simulink library "Navigation_Lib"  (R2014a)
settings: Solver=ode45  StartTime=0.0  StopTime=10.0  RelTol=1e-3
undefined symbols (not defined in the file or in its folder): DiscIntNeverNeededParam, gyro_x_offset, gyro_y_offset, gyro_z_offset
libraries: simulink x7, aerolibutil x5, vrlib x4, aerolibtransform2 x3, dspmtrx3 x2
(part 1 of 3)
settings Model: Creator=darenlee  LastModifiedBy=darenlee

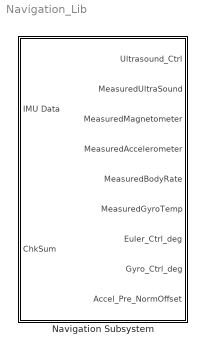
== system Navigation_Lib ==
  Navigation Subsystem : Subsystem  mask{TempProcessVariant=1, PI_YAW_CORRECT=[-0.9 -0.0001], D_YAW_CORRECT=0, P_GAIN_ROLLPITCH=-2, I_GAIN_ROLLPITCH=-0.01, ACCEL_OFFSET_X=0, ACCEL_OFFSET_Y=0, ACCEL_OFFSET_Z=0}
      mask prompts: TempProcessVariant "TempCondition"; PI_YAW_CORRECT "PI Gain  (Yaw Correction)"; D_YAW_CORRECT "D Gain (Yaw Correction)"; P_GAIN_ROLLPITCH "P Gain (RollPitch Correction)"; I_GAIN_ROLLPITCH "I Gain (RollPitch Correction)"; ACCEL_OFFSET_X "Accel Offset X"; ACCEL_OFFSET_Y "Accel Offset Y"; ACCEL_OFFSET_Z "Accel Offset Z"
      mask TypeOptions TempProcessVariant: 1 | 2
      mask DialogControl DescTextVar Prompt: Navigation Subsystem with Attitude Determination

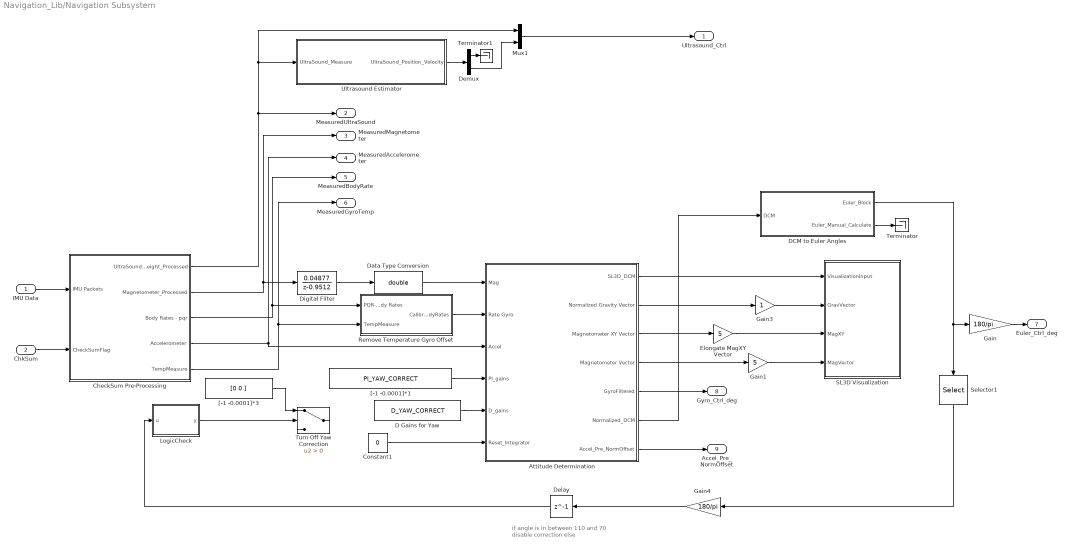
== system Navigation_Lib/Navigation Subsystem ==
  note: if angle is in between 110 and 70
      | disable correction
      | else
  IMU Data : Inport  OutDataTypeStr=Bus: IMU_Packets
  ChkSum : Inport  Port=2
  Attitude Determination : Subsystem
  CheckSum Pre-Processing : Subsystem
  Constant1 : Constant  Value=0
  D Gains for Yaw : Constant  Value=D_YAW_CORRECT
  DCM to Euler Angles : Subsystem
  Data Type Conversion : DataTypeConversion  OutDataTypeStr=double
  Delay : Delay  DelayLength=1  InitialCondition=0
  Demux : Demux  Outputs=2
  Digital Filter : DiscreteTransferFcn  Numerator=[0.04877]  Denominator=[1 -0.9512]  SampleTime=1/400
  Elongate MagXY Vector : Gain  Gain=5  OutDataTypeStr=double
  Gain : Gain  Gain=180/pi
  Gain1 : Gain  Gain=5  OutDataTypeStr=double
  Gain3 : Gain  OutDataTypeStr=double
  Gain4 : Gain  Gain=180/pi
  LogicCheck : MATLAB Function  TreatAsAtomicUnit=on
  Mux1 : Mux  Inputs=2
  Remove Temperature Gyro Offset : Subsystem  Variant=on  OverrideUsingVariant=TempProcessVariant==1
  SL3D Visualization : Subsystem
  Selector1 : Selector  IndexMode=Zero-based  InputPortWidth=3  Indices=2
  Terminator : Terminator
  Terminator1 : Terminator
  "Turn Off Yaw Correction " : Switch  Criteria=u2 > Threshold
  Ultrasound Estimator : Subsystem
  "[-1 -0.0001]*1" : Constant  Value=PI_YAW_CORRECT
  "[-1 -0.0001]*3" : Constant  Value=[0 0 ]
  Ultrasound_Ctrl : Outport
  MeasuredUltraSound : Outport  Port=2
  MeasuredMagnetometer : Outport  Port=3
  MeasuredAccelerometer : Outport  Port=4
  MeasuredBodyRate : Outport  Port=5
  MeasuredGyroTemp : Outport  Port=6
  Euler_Ctrl_deg : Outport  Port=7
  Gyro_Ctrl_deg : Outport  Port=8
  "Accel_Pre_NormOffset " : Outport  Port=9
  wires:
  DCM to Euler Angles/2(Euler_Manual_Calculate) -> Terminator/1
  "[-1 -0.0001]*1"/1 -> Attitude Determination/4(PI_gains)
  Remove Temperature Gyro Offset/1(Calibrated-BodyRates) -> Attitude Determination/2(Rate Gyro)
  D Gains for Yaw/1 -> Attitude Determination/5(D_gains)
  Gain4/1 -> Delay/1
  Selector1/1 -> Gain4/1
  LogicCheck/1(y) -> "Turn Off Yaw Correction "/2
  Delay/1 -> LogicCheck/1(u)
  "[-1 -0.0001]*3"/1 -> "Turn Off Yaw Correction "/1
  Attitude Determination/5(GyroFiltered) -> Gyro_Ctrl_deg/1
  Attitude Determination/3(" Magnetometer XY Vector") -> Elongate MagXY Vector/1
  Attitude Determination/4(Magnetometer Vector) -> Gain1/1
  Gain3/1 -> SL3D Visualization/2(GravVector)
  Attitude Determination/2(Normalized Gravity Vector) -> Gain3/1
  Constant1/1 -> Attitude Determination/6(Reset_Integrator)
  Elongate MagXY Vector/1 -> SL3D Visualization/3(MagXY)
  Gain1/1 -> SL3D Visualization/4(MagVector)
  Attitude Determination/1(SL3D_DCM) -> SL3D Visualization/1(VisualizationInput)
  Digital Filter/1 -> Data Type Conversion/1
  DCM to Euler Angles/1(Euler_Block) -> Gain/1, Selector1/1
  CheckSum Pre-Processing/5(TempMeasure) -> Remove Temperature Gyro Offset/2(TempMeasure), MeasuredGyroTemp/1
  CheckSum Pre-Processing/2(Magnetometer_Processed) -> Digital Filter/1, MeasuredMagnetometer/1
  CheckSum Pre-Processing/3(Body Rates - pqr) -> Remove Temperature Gyro Offset/1(PQR-Body Rates), MeasuredBodyRate/1
  CheckSum Pre-Processing/4(Accelerometer) -> Attitude Determination/3(Accel), MeasuredAccelerometer/1
  ChkSum/1 -> CheckSum Pre-Processing/2(CheckSumFlag)
  IMU Data/1 -> CheckSum Pre-Processing/1(IMU Packets)
  Attitude Determination/6("Normalized_DCM ") -> DCM to Euler Angles/1(DCM)
  Data Type Conversion/1 -> Attitude Determination/1(Mag)
  Attitude Determination/7(Accel_Pre_NormOffset) -> "Accel_Pre_NormOffset "/1
  Gain/1 -> Euler_Ctrl_deg/1
  CheckSum Pre-Processing/1(UltraSoundHeight_Processed) -> Ultrasound Estimator/1(UltraSound_Measure), Mux1/1, MeasuredUltraSound/1
  Mux1/1 -> Ultrasound_Ctrl/1
  Ultrasound Estimator/1("UltraSound_Position_Velocity ") -> Demux/1
  Demux/2 -> Mux1/2
  Demux/1 -> Terminator1/1

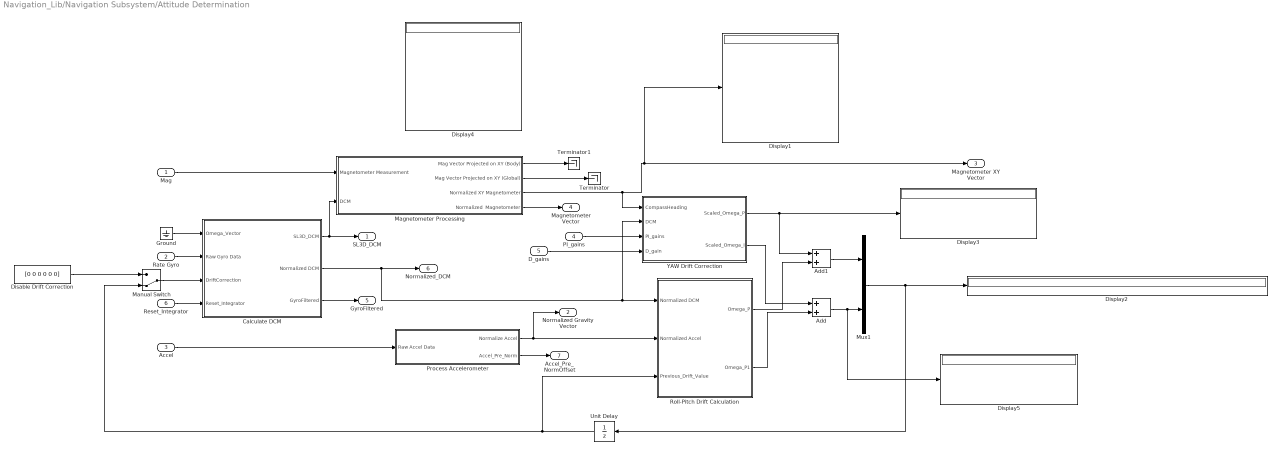
== system Navigation_Lib/Navigation Subsystem/Attitude Determination ==
  Mag : Inport  PortDimensions=3
  Rate Gyro : Inport  Port=2  PortDimensions=3
  Accel : Inport  Port=3  OutDataTypeStr=uint16
  PI_gains : Inport  Port=4
  D_gains : Inport  Port=5
  Reset_Integrator : Inport  Port=6
  Add : Sum
  Add1 : Sum
  Calculate DCM : Subsystem
  Disable Drift Correction : Constant  Value=[0 0 0 0 0 0]
  Display{1..5} (5 alike) : Display
  Ground : Ground
  Magnetometer Processing : Subsystem
  Manual Switch : ManualSwitch  CurrentSetting=0
  Mux1 : Mux  Inputs=2
  Process Accelerometer : Subsystem
  Roll-Pitch Drift Calculation : Subsystem
  Terminator : Terminator
  Terminator1 : Terminator
  Unit Delay : UnitDelay  SampleTime=-1
  YAW Drift Correction : Subsystem  TreatAsAtomicUnit=on
  SL3D_DCM : Outport
  Normalized Gravity Vector : Outport  Port=2
  " Magnetometer XY Vector" : Outport  Port=3
  Magnetometer Vector : Outport  Port=4
  GyroFiltered : Outport  Port=5
  "Normalized_DCM " : Outport  Port=6
  Accel_Pre_NormOffset : Outport  Port=7
  wires:
  Calculate DCM/2(Normalized DCM) -> YAW Drift Correction/2(DCM), Roll-Pitch Drift Calculation/1(Normalized DCM), "Normalized_DCM "/1
  Manual Switch/1 -> Calculate DCM/3(DriftCorrection)
  Process Accelerometer/1(Normalize Accel) -> Normalized Gravity Vector/1, Roll-Pitch Drift Calculation/2(Normalized Accel)
  D_gains/1 -> YAW Drift Correction/4(D_gain)
  Magnetometer Processing/1(Mag Vector Projected on XY (Body)) -> Terminator1/1
  Disable Drift Correction/1 -> Manual Switch/1
  Accel/1 -> Process Accelerometer/1(Raw Accel Data)
  Process Accelerometer/2(Accel_Pre_Norm) -> Accel_Pre_NormOffset/1
  Mag/1 -> Magnetometer Processing/1(Magnetometer Measurement)
  Magnetometer Processing/2(Mag Vector Projected on XY (Global)) -> Terminator/1
  Calculate DCM/1(SL3D_DCM) -> SL3D_DCM/1, Magnetometer Processing/2(DCM)
  Add/1 -> Display5/1, Mux1/2
  Add1/1 -> Mux1/1
  Roll-Pitch Drift Calculation/1(Omega_P) -> Add1/2
  Roll-Pitch Drift Calculation/2(Omega_P1) -> Add/2
  PI_gains/1 -> YAW Drift Correction/3(PI_gains)
  Magnetometer Processing/3(Normalized XY Magnetometer) -> Display1/1, " Magnetometer XY Vector"/1, YAW Drift Correction/1(CompassHeading)
  Magnetometer Processing/4(Normalized  Magnetometer) -> Magnetometer Vector/1
  YAW Drift Correction/1(Scaled_Omega_P) -> Display3/1, Add1/1
  YAW Drift Correction/2(Scaled_Omega_I) -> Add/1
  Reset_Integrator/1 -> Calculate DCM/4("Reset_Integrator ")
  Calculate DCM/3(GyroFiltered) -> GyroFiltered/1
  Mux1/1 -> Unit Delay/1, Display2/1
  Rate Gyro/1 -> Calculate DCM/2(Raw Gyro Data)
  Unit Delay/1 -> Manual Switch/2, Roll-Pitch Drift Calculation/3(Previous_Drift_Value)
  Ground/1 -> Calculate DCM/1(Omega_Vector)

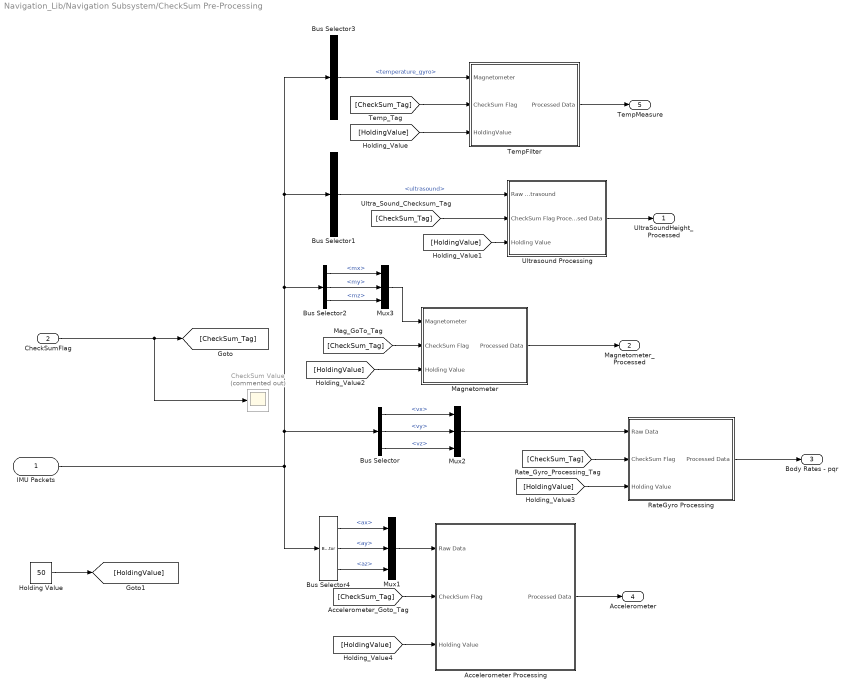
== system Navigation_Lib/Navigation Subsystem/CheckSum Pre-Processing ==
  IMU Packets : Inport
  CheckSumFlag : Inport  Port=2
  Accelerometer Processing : Subsystem
  Bus Selector : BusSelector  OutputSignals=vx,vy,vz
  Bus Selector1 : BusSelector  OutputSignals=ultrasound
  Bus Selector2 : BusSelector  OutputSignals=mx,my,mz
  Bus Selector3 : BusSelector  OutputSignals=temperature_gyro
  Bus Selector4 : BusSelector  OutputSignals=ax,ay,az
  CheckSum Value : Scope  Commented=on
      settings: YMin=0  YMax=2500  SaveName=CheckSum
  Holding Value : Constant  Value=50
  Magnetometer : Subsystem
  Mux1 : Mux  Inputs=3
  Mux2 : Mux  Inputs=3
  Mux3 : Mux  Inputs=3
  RateGyro Processing : Subsystem
  TempFilter : Subsystem
  Ultrasound Processing : Subsystem
  UltraSoundHeight_Processed : Outport
  Magnetometer_Processed : Outport  Port=2
  Body Rates - pqr : Outport  Port=3
  Accelerometer : Outport  Port=4
  TempMeasure : Outport  Port=5
  wires:
  Holding Value/1 -> [HoldingValue]
  [HoldingValue] -> Accelerometer Processing/3(Holding Value)
  [HoldingValue] -> RateGyro Processing/3(Holding Value)
  [HoldingValue] -> Magnetometer/3(Holding Value)
  [HoldingValue] -> Ultrasound Processing/3(Holding Value)
  [HoldingValue] -> TempFilter/3(HoldingValue)
  [CheckSum_Tag] -> TempFilter/2(CheckSum Flag)
  TempFilter/1(Processed Data) -> TempMeasure/1
  Bus Selector3/1 -> TempFilter/1(Magnetometer)  "<temperature_gyro>"
  Bus Selector/3 -> Mux2/3  "<vz>"
  Bus Selector/2 -> Mux2/2  "<vy>"
  Bus Selector/1 -> Mux2/1  "<vx>"
  Ultrasound Processing/1(Processed Data) -> UltraSoundHeight_Processed/1
  [CheckSum_Tag] -> Accelerometer Processing/2(CheckSum Flag)
  Magnetometer/1(Processed Data) -> Magnetometer_Processed/1
  [CheckSum_Tag] -> Magnetometer/2(CheckSum Flag)
  Mux3/1 -> Magnetometer/1(Magnetometer)
  Bus Selector2/3 -> Mux3/3  "<mz>"
  Bus Selector2/2 -> Mux3/2  "<my>"
  Bus Selector2/1 -> Mux3/1  "<mx>"
  RateGyro Processing/1(Processed Data) -> Body Rates - pqr/1
  [CheckSum_Tag] -> RateGyro Processing/2(CheckSum Flag)
  Mux2/1 -> RateGyro Processing/1(Raw Data)
  Accelerometer Processing/1(Processed Data) -> Accelerometer/1
  [CheckSum_Tag] -> Ultrasound Processing/2(CheckSum Flag)
  Mux1/1 -> Accelerometer Processing/1(Raw Data)
  Bus Selector4/3 -> Mux1/3  "<az>"
  Bus Selector4/2 -> Mux1/2  "<ay>"
  Bus Selector4/1 -> Mux1/1  "<ax>"
  IMU Packets/1 -> Bus Selector4/1, Bus Selector2/1, Bus Selector1/1, Bus Selector3/1, Bus Selector/1
  CheckSumFlag/1 -> CheckSum Value/1, [CheckSum_Tag]
  Bus Selector1/1 -> Ultrasound Processing/1(Raw Ultrasound)  "<ultrasound>"

== system Navigation_Lib/Navigation Subsystem/DCM to Euler Angles ==
  note: Euler Rotation Order:
      | With the camera facing towards you
      | ______________
      |       Camera          |
      | 1                    2    |
      |                             |
      | 3                    4    |
      | ______________|
      |
      | Rotation
      |
      | Roll+ , increase 2+4
      | Roll - , increase 1 3
      |
      | Pitch+ , increaes 1+2
      | Pitch- , increase 3+4
  DCM : Inport
  Constant2 : Constant  Value=[1 0 0]
  Direction Cosine Matrix to Rotation Angles : aerolibtransform2/Direction Cosine Matrix to Rotation Angles  rotationOrder=XYZ  lim=Default
      settings: AttributesFormatString=Rotation Order: %<rotationOrder>
  EulerAnglesCalculation : Subsystem  TreatAsAtomicUnit=on
  Product : Product  Multiplication=Matrix(*)
  VectorTrace : Scope
      settings: SaveName=RotationVectorTrace
  Euler_Block : Outport
  Euler_Manual_Calculate : Outport  Port=2
  wires:
  Product/1 -> VectorTrace/1
  Constant2/1 -> Product/2
  Direction Cosine Matrix to Rotation Angles/1 -> Euler_Block/1
  EulerAnglesCalculation/1(Euler Angles) -> Euler_Manual_Calculate/1
  DCM/1 -> EulerAnglesCalculation/1(DCM), Product/1, Direction Cosine Matrix to Rotation Angles/1

== system Navigation_Lib/Navigation Subsystem/Remove Temperature Gyro Offset ==
  note: 1) Only subsystems can be added as variant choices at this level
      | 2) Blocks cannot be connected at this level as connectivity is
      | automatically determined at simulation, based on the active variant
  PQR-Body Rates : Inport
  TempMeasure : Inport  Port=2
  TemperatureOffset (home_330453) : Subsystem  VariantControl=TempProcessVariant==1
  TemperatureOffset (work_255725) : Subsystem  VariantControl=TempProcessVariant==2
  Calibrated-BodyRates : Outport

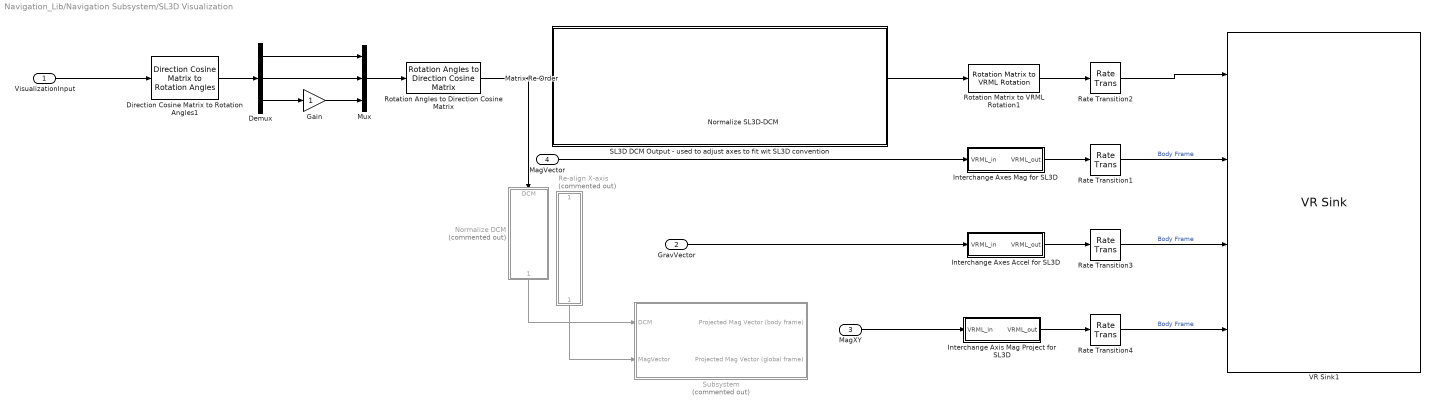
== system Navigation_Lib/Navigation Subsystem/SL3D Visualization ==
  VisualizationInput : Inport
  GravVector : Inport  Port=2
  MagXY : Inport  Port=3
  MagVector : Inport  Port=4
  Demux : Demux  Outputs=3
  Direction Cosine Matrix to Rotation Angles1 : aerolibtransform2/Direction Cosine Matrix to Rotation Angles  rotationOrder=XYZ  lim=ZeroR3
      settings: AttributesFormatString=Rotation Order: %<rotationOrder>
  Gain : Gain  OutDataTypeStr=Inherit: Same as input
  "Interchange Axes Accel for SL3D " : Subsystem
  "Interchange Axes Mag for SL3D " : Subsystem
  Interchange Axis Mag Project for SL3D : Subsystem
  Matrix Re-Order : MATLAB Function  TreatAsAtomicUnit=on
  Mux : Mux  Inputs=3
  Normalize DCM : Subsystem  Commented=on  TreatAsAtomicUnit=on
  Normalize SL3D-DCM : Subsystem  TreatAsAtomicUnit=on
  Rate Transition{1..4} (4 alike) : RateTransition
  Re-align X-axis : Subsystem  Commented=on
  Rotation Angles to Direction Cosine Matrix : aerolibtransform2/Rotation Angles to Direction Cosine Matrix  rotationOrder=XYZ
  Rotation Matrix to VRML Rotation1 : vrlib/Utilities/Rotation Matrix to VRML Rotation  maxzero=1e-12
  SL3D DCM Output - used to adjust axes to fit wit SL3D convention : Subsystem
  Subsystem : Subsystem  Commented=on
  VR Sink1 : vrlib/VR Sink  InstantiateOnLoad=on  SampleTime=0.02  ViewEnable=on  RemoteChange=off  RemoteView=off  FieldsWritten=Plane.rotation.4.1.1.double#mag_point.translation.3.1.1.double#grav_point.translation.3.1.1.double#mag_projection_point.translation.3.1.1.double  WorldFileName=AR_Drone_Visualization.WRL  AutoView=off  VideoDimensions=[]  AllowVariableSize=off
  wires:
  MagXY/1 -> Interchange Axis Mag Project for SL3D/1(VRML_in)
  Re-align X-axis/1(MagVectorOut) -> Subsystem/2(MagVector)
  Normalize DCM/1(DCM_normalized) -> Subsystem/1(DCM)
  Rate Transition2/1 -> VR Sink1/1
  Rate Transition1/1 -> VR Sink1/2  "Body Frame"
  Rate Transition3/1 -> VR Sink1/3  "Body Frame"
  Rate Transition4/1 -> VR Sink1/4  "Body Frame"
  Interchange Axis Mag Project for SL3D/1(VRML_out) -> Rate Transition4/1
  Rotation Angles to Direction Cosine Matrix/1 -> Normalize DCM/1(DCM), Matrix Re-Order/1(M_in)
  MagVector/1 -> "Interchange Axes Mag for SL3D "/1(VRML_in)
  "Interchange Axes Mag for SL3D "/1(VRML_out) -> Rate Transition1/1
  Normalize SL3D-DCM/1(DCM_normalized) -> Rotation Matrix to VRML Rotation1/1
  Matrix Re-Order/1(M_out) -> Normalize SL3D-DCM/1(DCM)
  GravVector/1 -> "Interchange Axes Accel for SL3D "/1(VRML_in)
  "Interchange Axes Accel for SL3D "/1(VRML_out) -> Rate Transition3/1
  Rotation Matrix to VRML Rotation1/1 -> Rate Transition2/1
  Direction Cosine Matrix to Rotation Angles1/1 -> Demux/1
  Demux/1 -> Mux/1
  Demux/2 -> Mux/2
  Demux/3 -> Gain/1
  Gain/1 -> Mux/3
  Mux/1 -> Rotation Angles to Direction Cosine Matrix/1
  VisualizationInput/1 -> Direction Cosine Matrix to Rotation Angles1/1

== system Navigation_Lib/Navigation Subsystem/Ultrasound Estimator ==
  UltraSound_Measure : Inport
  Kalman Tracker : MATLAB Function  TreatAsAtomicUnit=on
  Unit Delay1 : UnitDelay  InitialCondition=[0 0 ]  SampleTime=-1
  Unit Delay2 : UnitDelay  InitialCondition=eye(2)  SampleTime=-1
  "UltraSound_Position_Velocity " : Outport
  wires:
  Kalman Tracker/2(covariance_correction) -> Unit Delay2/1
  Kalman Tracker/1(state_correction) -> Unit Delay1/1
  UltraSound_Measure/1 -> Kalman Tracker/1(UltraSoundMeasure)
  Unit Delay2/1 -> Kalman Tracker/2(covariance_correction_input)
  Unit Delay1/1 -> "UltraSound_Position_Velocity "/1, Kalman Tracker/3(state_correction_input)

== system Navigation_Lib/Navigation Subsystem/Attitude Determination/Calculate DCM ==
  Omega_Vector : Inport
  Raw Gyro Data : Inport  Port=2
  DriftCorrection : Inport  Port=3
  "Reset_Integrator " : Inport  Port=4
  Calculate Deltas : Subsystem
  Matrix Re-Order : MATLAB Function  Commented=through  TreatAsAtomicUnit=on
  Normalize DCM : Subsystem  TreatAsAtomicUnit=on
  Normalize SL3D-DCM : Subsystem  Commented=through  TreatAsAtomicUnit=on
  Process Raw Rate Gyro Data : Subsystem
  SL3D DCM Output - used to adjust axes to fit wit SL3D convention : Subsystem
  Terminator : Terminator
  Update DCM : Subsystem  TreatAsAtomicUnit=on  VariantControl=UncorrectedMode
  deg2rad : Gain  Gain=pi/180
  SL3D_DCM : Outport
  Normalized DCM : Outport  Port=2
  GyroFiltered : Outport  Port=3
  wires:
  Process Raw Rate Gyro Data/1(Processed Data) -> deg2rad/1
  deg2rad/1 -> Calculate Deltas/1(Adjusted)
  Calculate Deltas/2(Omega) -> GyroFiltered/1, Terminator/1
  Raw Gyro Data/1 -> Process Raw Rate Gyro Data/1(Raw Data)
  Update DCM/1(DCM Matrix) -> Matrix Re-Order/1(M_in), Normalize DCM/1(DCM)
  Normalize DCM/1(DCM_normalized) -> Normalized DCM/1
  Omega_Vector/1 -> Update DCM/1(Omega vector)
  Calculate Deltas/1(Gyro_Vector(G_Dt)) -> Update DCM/2(Gyro vector)
  Matrix Re-Order/1(M_out) -> Normalize SL3D-DCM/1(DCM)
  Normalize SL3D-DCM/1(DCM_normalized) -> SL3D_DCM/1
  DriftCorrection/1 -> Calculate Deltas/2(DriftCorrection)
  "Reset_Integrator "/1 -> Update DCM/3("Reset_Integrator ")

== system Navigation_Lib/Navigation Subsystem/Attitude Determination/Magnetometer Processing ==
  Magnetometer Measurement : Inport
  DCM : Inport  Port=2
  Magnetometer Heading Calculation : Subsystem
  Normalize Vector : vrlib/Utilities/Normalize Vector  maxzero=0
  Normalize Vector1 : vrlib/Utilities/Normalize Vector  maxzero=0
  Process Raw Mag Data : Subsystem  Variant=on  OverrideUsingVariant=TempProcessVariant==1
  Re-align X-axis : Subsystem
  Mag Vector Projected on XY (Body) : Outport
  Mag Vector Projected on XY (Global) : Outport  Port=2
  Normalized XY Magnetometer : Outport  Port=3
  Normalized  Magnetometer : Outport  Port=4
  wires:
  Magnetometer Heading Calculation/2(Projected Mag Vector (global frame)) -> Mag Vector Projected on XY (Global)/1
  Normalize Vector/1 -> Normalized  Magnetometer/1, Re-align X-axis/1(MagVector)
  Process Raw Mag Data/1(MagVector) -> Normalize Vector/1
  Re-align X-axis/1(MagVectorOut) -> Magnetometer Heading Calculation/1(MagVector)
  Magnetometer Measurement/1 -> Process Raw Mag Data/1(Magnetometer)
  Magnetometer Heading Calculation/1(Projected Mag Vector (body frame)) -> Normalize Vector1/1
  DCM/1 -> Magnetometer Heading Calculation/2(DCM)
  Normalize Vector1/1 -> Normalized XY Magnetometer/1, Mag Vector Projected on XY (Body)/1

== system Navigation_Lib/Navigation Subsystem/Attitude Determination/Process Accelerometer ==
  Raw Accel Data : Inport
  Accelerometer Correction Offset : Subsystem
  Accelerometer Neutral Gain and Offset : Subsystem
  Low Pass Filter : Subsystem
  Normalize Accel : Outport
  Accel_Pre_Norm : Outport  Port=2
  wires:
  Raw Accel Data/1 -> Accelerometer Neutral Gain and Offset/1(Raw Accel Data)
  Accelerometer Neutral Gain and Offset/2(Accel_Pre_Norm) -> Accel_Pre_Norm/1
  Accelerometer Neutral Gain and Offset/1(Processed Accel Data) -> Accelerometer Correction Offset/1(Accelerometer)
  Accelerometer Correction Offset/1(OffsetCorrection) -> Low Pass Filter/1(Offset Accel)
  Low Pass Filter/1(Filtered Accel) -> Normalize Accel/1

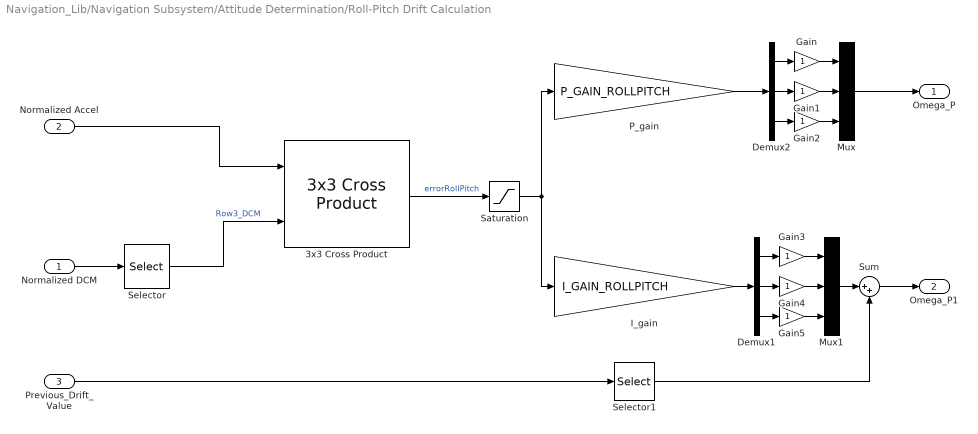
== system Navigation_Lib/Navigation Subsystem/Attitude Determination/Roll-Pitch Drift Calculation ==
  Normalized DCM : Inport
  Normalized Accel : Inport  Port=2
  Previous_Drift_Value : Inport  Port=3
  3x3 Cross Product : aerolibutil/3x3 Cross Product
  Demux1 : Demux  Outputs=3
  Demux2 : Demux  Outputs=3
  Gain{,1..5} (6 alike) : Gain  OutDataTypeStr=Inherit: Same as input
  I_gain : Gain  Gain=I_GAIN_ROLLPITCH
  Mux : Mux  Inputs=3
  Mux1 : Mux  Inputs=3
  P_gain : Gain  Gain=P_GAIN_ROLLPITCH
  Saturation : Saturate  UpperLimit=50  LowerLimit=-50
      settings: AttributesFormatString=%<LowerLimit> to %<UpperLimit>
  Selector : Selector  NumberOfDimensions=2  IndexMode=Zero-based  InputPortWidth=3,3  IndexOptions=Index vector (dialog),Select all  Indices=2,[1:3]  OutputSizes=1,1
  Selector1 : Selector  IndexMode=Zero-based  InputPortWidth=6  Indices=[3:5]
  Sum : Sum  Inputs=|++
  Omega_P : Outport
  Omega_P1 : Outport  Port=2
  wires:
  Selector/1 -> 3x3 Cross Product/2  "Row3_DCM"
  3x3 Cross Product/1 -> Saturation/1  "errorRollPitch"
  Normalized DCM/1 -> Selector/1
  Normalized Accel/1 -> 3x3 Cross Product/1
  Saturation/1 -> P_gain/1, I_gain/1
  Sum/1 -> Omega_P1/1
  Previous_Drift_Value/1 -> Selector1/1
  Selector1/1 -> Sum/2
  Demux2/1 -> Gain/1
  Gain/1 -> Mux/1
  Demux2/2 -> Gain1/1
  Gain1/1 -> Mux/2
  Demux2/3 -> Gain2/1
  Gain2/1 -> Mux/3
  P_gain/1 -> Demux2/1
  Mux/1 -> Omega_P/1
  Demux1/1 -> Gain3/1
  Gain3/1 -> Mux1/1
  Demux1/2 -> Gain4/1
  Gain4/1 -> Mux1/2
  Demux1/3 -> Gain5/1
  Gain5/1 -> Mux1/3
  I_gain/1 -> Demux1/1
  Mux1/1 -> Sum/1

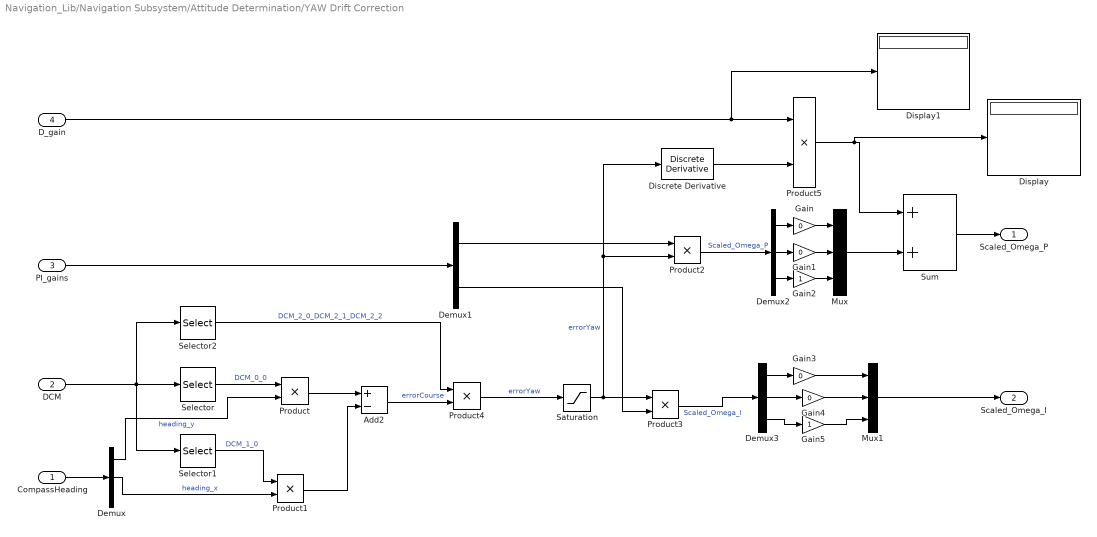
== system Navigation_Lib/Navigation Subsystem/Attitude Determination/YAW Drift Correction ==
  CompassHeading : Inport
  DCM : Inport  Port=2
  PI_gains : Inport  Port=3
  D_gain : Inport  Port=4
  Add2 : Sum  Inputs=+-
  Demux : Demux  Outputs=3
  Demux1 : Demux  Outputs=2
  Demux2 : Demux  Outputs=3
  Demux3 : Demux  Outputs=3
  Discrete Derivative : simulink/Discrete/Discrete Derivative  gainval=1.0  ICPrevScaledInput=0.01  InputProcessing=Inherited  OutMin=[]  OutMax=[]  OutDataType=fixdt(1, 16)  OutScaling=2^-10  DoSatur=off
  Display : Display
  Display1 : Display
  Gain{,1,3..4} (4 alike) : Gain  Gain=0  OutDataTypeStr=Inherit: Same as input
  Gain2 : Gain  OutDataTypeStr=Inherit: Same as input
  Gain5 : Gain  OutDataTypeStr=Inherit: Same as input
  Mux : Mux  Inputs=3
  Mux1 : Mux  Inputs=3
  Product{,1..5} (6 alike) : Product  RndMeth=Zero
  Saturation : Saturate  UpperLimit=50  LowerLimit=-50
      settings: AttributesFormatString=%<LowerLimit> to %<UpperLimit>
  Selector : Selector  NumberOfDimensions=2  IndexMode=Zero-based  InputPortWidth=3  IndexOptions=Index vector (dialog),Index vector (dialog)  Indices=0,0  OutputSizes=1,1
  Selector1 : Selector  NumberOfDimensions=2  IndexMode=Zero-based  InputPortWidth=3  IndexOptions=Index vector (dialog),Index vector (dialog)  Indices=1,0  OutputSizes=1,1
  Selector2 : Selector  NumberOfDimensions=2  IndexMode=Zero-based  InputPortWidth=3  IndexOptions=Index vector (dialog),Select all  Indices=2,0  OutputSizes=1,1
  Sum : Sum
  Scaled_Omega_P : Outport  OutputWhenDisabled=reset  InitialOutput=[0 0 0]
  Scaled_Omega_I : Outport  Port=2  OutputWhenDisabled=reset  InitialOutput=[0 0 0]
  wires:
  Product4/1 -> Saturation/1  "errorYaw"
  Selector2/1 -> Product4/1  "DCM_2_0_DCM_2_1_DCM_2_2"
  Product1/1 -> Add2/2
  Product/1 -> Add2/1
  Demux/1 -> Product/2  "heading_y"
  Demux/2 -> Product1/2  "heading_x"
  CompassHeading/1 -> Demux/1
  Selector1/1 -> Product1/1  "DCM_1_0"
  Selector/1 -> Product/1  "DCM_0_0"
  DCM/1 -> Selector2/1, Selector1/1, Selector/1
  Add2/1 -> Product4/2  "errorCourse"
  Saturation/1 -> Product2/2, Discrete Derivative/1, Product3/1  "errorYaw"
  Product2/1 -> Demux2/1  "Scaled_Omega_P"
  Product3/1 -> Demux3/1  "Scaled_Omega_I"
  Demux1/1 -> Product2/1
  Demux1/2 -> Product3/2
  PI_gains/1 -> Demux1/1
  Mux1/1 -> Scaled_Omega_I/1
  Demux2/1 -> Gain/1
  Gain/1 -> Mux/1
  Demux2/2 -> Gain1/1
  Gain1/1 -> Mux/2
  Demux2/3 -> Gain2/1
  Gain2/1 -> Mux/3
  Demux3/1 -> Gain3/1
  Demux3/2 -> Gain4/1
  Demux3/3 -> Gain5/1
  Gain3/1 -> Mux1/1
  Gain4/1 -> Mux1/2
  Gain5/1 -> Mux1/3
  Discrete Derivative/1 -> Product5/2
  D_gain/1 -> Display1/1, Product5/1
  Product5/1 -> Display/1, Sum/1
  Mux/1 -> Sum/2
  Sum/1 -> Scaled_Omega_P/1

== system Navigation_Lib/Navigation Subsystem/CheckSum Pre-Processing/Accelerometer Processing ==
  Raw Data : Inport
  CheckSum Flag : Inport  Port=2
  Holding Value : Inport  Port=3
  Calculate Accel Data : Subsystem  Commented=through
  CheckSum Correction : Subsystem
  Processed Data : Outport
  wires:
  Holding Value/1 -> CheckSum Correction/3(Holding Value)
  Calculate Accel Data/1(Processed Accel Data) -> CheckSum Correction/1(CalculatedData)
  CheckSum Correction/1(Pre-Processed Height) -> Processed Data/1
  Raw Data/1 -> Calculate Accel Data/1(Raw Accel Data)
  CheckSum Flag/1 -> CheckSum Correction/2(CheckSumFlag)

== system Navigation_Lib/Navigation Subsystem/CheckSum Pre-Processing/Magnetometer ==
  Magnetometer : Inport
  CheckSum Flag : Inport  Port=2
  Holding Value : Inport  Port=3
  CheckSum Correction : Subsystem
  Display : Display
  Process Raw Mag Data : Subsystem  Commented=through
  Processed Data : Outport
  wires:
  Holding Value/1 -> CheckSum Correction/3(Holding Value)
  Process Raw Mag Data/1(ProcessedData) -> CheckSum Correction/1(CalculatedData)
  Magnetometer/1 -> Process Raw Mag Data/1(Magnetometer)
  CheckSum Correction/1(Pre-Processed Data) -> Processed Data/1, Display/1
  CheckSum Flag/1 -> CheckSum Correction/2(CheckSumFlag)

== system Navigation_Lib/Navigation Subsystem/CheckSum Pre-Processing/RateGyro Processing ==
  Raw Data : Inport
  CheckSum Flag : Inport  Port=2
  Holding Value : Inport  Port=3
  CheckSum Correction : Subsystem
  Process Data : Subsystem  Commented=through
  Processed Data : Outport
  wires:
  Holding Value/1 -> CheckSum Correction/3(Holding Value)
  Process Data/1(Processed Data) -> CheckSum Correction/1(CalculatedData)
  Raw Data/1 -> Process Data/1(Raw Data)
  CheckSum Correction/1(Pre-Processed Height) -> Processed Data/1
  CheckSum Flag/1 -> CheckSum Correction/2(CheckSumFlag)

== system Navigation_Lib/Navigation Subsystem/CheckSum Pre-Processing/TempFilter ==
  Magnetometer : Inport
  CheckSum Flag : Inport  Port=2
  HoldingValue : Inport  Port=3
  CheckSum Correction : Subsystem
  Display : Display
  Process Raw Mag Data : Subsystem  Commented=through
  Processed Data : Outport
  wires:
  HoldingValue/1 -> CheckSum Correction/3(Holding Value)
  Process Raw Mag Data/1(ProcessedData) -> CheckSum Correction/1(CalculatedData)
  Magnetometer/1 -> Process Raw Mag Data/1(Magnetometer)
  CheckSum Correction/1(Pre-Processed Data) -> Processed Data/1, Display/1
  CheckSum Flag/1 -> CheckSum Correction/2(CheckSumFlag)

== system Navigation_Lib/Navigation Subsystem/CheckSum Pre-Processing/Ultrasound Processing ==
  note: '192.168.1.1' 1 17725
  Raw Ultrasound : Inport
  CheckSum Flag : Inport  Port=2
  Holding Value : Inport  Port=3
  CheckSum Correction : Subsystem
  Data Type Conversion1 : DataTypeConversion
  Delay1 : Delay  DelayLength=1  InitialCondition=0
  Display : Display
  Height Calculation : MATLAB Function  TreatAsAtomicUnit=on
  Saturation1 : Saturate  UpperLimit=100e3  LowerLimit=0
  Processed Data : Outport
  wires:
  Holding Value/1 -> CheckSum Correction/3(Holding Value)
  Saturation1/1 -> Processed Data/1
  CheckSum Correction/1(Pre-Processed Height) -> Saturation1/1, Display/1
  CheckSum Flag/1 -> CheckSum Correction/2(CheckSumFlag)
  Height Calculation/1(y) -> CheckSum Correction/1(CalculatedData)
  Raw Ultrasound/1 -> Data Type Conversion1/1
  Height Calculation/2(prev_good_height) -> Delay1/1
  Data Type Conversion1/1 -> Height Calculation/1(u)
  Delay1/1 -> Height Calculation/2(z_1)

== system Navigation_Lib/Navigation Subsystem/DCM to Euler Angles/EulerAnglesCalculation ==
  DCM : Inport
  Demux : Demux  Outputs=2
  Demux1 : Demux  Outputs=2
  Gain : Gain  Gain=-1
  Gain1 : Gain  OutDataTypeStr=Inherit: Same as input
  Mux : Mux  Inputs=3
  Selector : Selector  NumberOfDimensions=2  IndexMode=Zero-based  InputPortWidth=3  IndexOptions=Index vector (dialog),Index vector (dialog)  Indices=2,0  OutputSizes=1,1
  Selector1 : Selector  NumberOfDimensions=2  IndexMode=Zero-based  InputPortWidth=3  IndexOptions=Index vector (dialog),Index vector (dialog)  Indices=2,[1 2]  OutputSizes=1,1
  Selector2 : Selector  NumberOfDimensions=2  IndexMode=Zero-based  InputPortWidth=3  IndexOptions=Index vector (dialog),Index vector (dialog)  Indices=[1 0],0  OutputSizes=1,1
  Trigonometric Function : Trigonometry  Operator=asin
  Trigonometric Function1 : Trigonometry  Operator=atan2
  Trigonometric Function2 : Trigonometry  Operator=atan2
  Euler Angles : Outport  InitialOutput=[0 0 0]
  wires:
  Gain1/1 -> Mux/3
  DCM/1 -> Selector1/1, Selector2/1, Selector/1
  Selector/1 -> Gain/1  "DCM_2_0"
  Gain/1 -> Trigonometric Function/1
  Trigonometric Function/1 -> Mux/2  "pitch"
  Selector1/1 -> Demux/1  "DCM_2_1_DCM_2_2"
  Demux/1 -> Trigonometric Function1/1
  Demux/2 -> Trigonometric Function1/2
  Trigonometric Function1/1 -> Mux/1  "roll"
  Trigonometric Function2/1 -> Gain1/1  "yaw"
  Selector2/1 -> Demux1/1  "DCM_1_0_DCM_0_0"
  Mux/1 -> Euler Angles/1
  Demux1/1 -> Trigonometric Function2/1
  Demux1/2 -> Trigonometric Function2/2

== system Navigation_Lib/Navigation Subsystem/Remove Temperature Gyro Offset/TemperatureOffset (home_330453) ==
  note: Yaw looks off
      |
      | Linear model Poly2:
      |      f(x) = p1*x^2 + p2*x + p3
      | Coefficients (with 95% confidence bounds):
      |        p1 =      0.2212  (0.2178, 0.2246)
      |        p2 =      -20.02  (-20.33, -19.71)
      |        p3 =       449.6  (442.4, 456.8)
  PQR-Body Rates : Inport
  TempMeasure : Inport  Port=2
  Convert to Celcius : Subsystem
  Data Type Conversion : DataTypeConversion
  Demux : Demux  Outputs=3
  Mux : Mux  Inputs=3
  Mux1 : Mux  Inputs=2
  Mux2 : Mux  Inputs=2
  Mux3 : Mux  Inputs=2
  Scope : Scope  NumInputPorts=3
      settings: ShowLegends=on  YMin=-10~-4~-4  YMax=120~11~14  SaveName=TempOffsetCorrect
  Sum1 : Sum  Inputs=|+-
  Sum2 : Sum  Inputs=|+-
  Sum3 : Sum  Inputs=|+-
  Temperature Correct Pitch : Subsystem  Commented=through
  Temperature Correct Pitch1 : Subsystem
  Temperature Correct Roll : Subsystem  Commented=through
  Temperature Correct Roll1 : Subsystem
  Temperature Correct Yaw : Subsystem  Commented=through
  Temperature Correct Yaw1 : Subsystem  Commented=through
  Calibrated-BodyRates : Outport
  wires:
  Temperature Correct Yaw1/1(Offset Correct) -> Sum3/2
  Temperature Correct Pitch1/1(Offset Correct) -> Sum2/2
  Temperature Correct Roll1/1(Offset Correct) -> Sum1/2
  Convert to Celcius/1(Out1) -> Temperature Correct Roll/1(Temp), Temperature Correct Pitch/1(Temp), Temperature Correct Yaw/1(Temp)
  TempMeasure/1 -> Convert to Celcius/1(In1)
  Temperature Correct Yaw/1(Offset Correct) -> Temperature Correct Yaw1/1(Temp)
  Temperature Correct Pitch/1(Offset Correct) -> Temperature Correct Pitch1/1(Temp)
  Temperature Correct Roll/1(Offset Correction) -> Temperature Correct Roll1/1(Temp)
  Mux3/1 -> Scope/3
  Mux2/1 -> Scope/2
  Mux1/1 -> Scope/1
  Sum2/1 -> Mux/2, Mux2/2  "Corrected Wy"
  Data Type Conversion/1 -> Calibrated-BodyRates/1
  Mux/1 -> Data Type Conversion/1
  PQR-Body Rates/1 -> Demux/1
  Demux/1 -> Sum1/1, Mux1/1  "Uncorrected Wx"
  Sum1/1 -> Mux/1, Mux1/2  "Corrected Wx"
  Demux/3 -> Sum3/1, Mux3/1  "Uncorrected Wz"
  Demux/2 -> Sum2/1, Mux2/1  "Uncorrected Wy"
  Sum3/1 -> Mux/3, Mux3/2  "Corrected Wz"

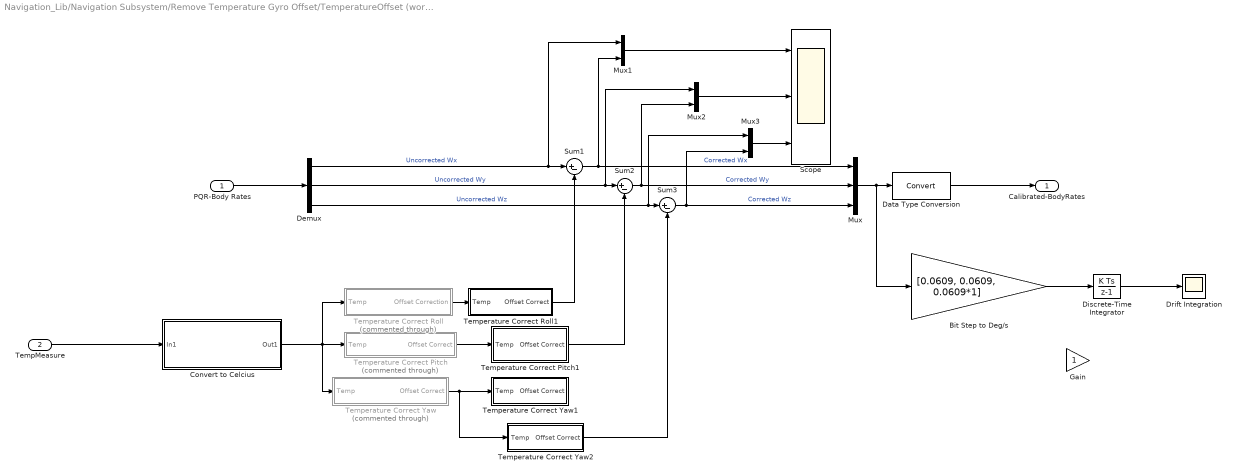
== system Navigation_Lib/Navigation Subsystem/Remove Temperature Gyro Offset/TemperatureOffset (work_255725) ==
  PQR-Body Rates : Inport
  TempMeasure : Inport  Port=2
  Bit Step to Deg/s : Gain  Gain=[0.0609, 0.0609, 0.0609*1]
  Convert to Celcius : Subsystem
  Data Type Conversion : DataTypeConversion
  Demux : Demux  Outputs=3
  Discrete-Time Integrator : DiscreteIntegrator  SampleTime=-1  ICPrevOutput=DiscIntNeverNeededParam  ICPrevScaledInput=DiscIntNeverNeededParam
  Drift Integration : Scope
      settings: YMin=0  YMax=2200  SaveName=ScopeData2
  Gain : Gain
  Mux : Mux  Inputs=3
  Mux1 : Mux  Inputs=2
  Mux2 : Mux  Inputs=2
  Mux3 : Mux  Inputs=2
  Scope : Scope  NumInputPorts=3
      settings: ShowLegends=on  YMin=-10~-22.5~-15  YMax=120~35~65  SaveName=TempOffsetCorrect
  Sum1 : Sum  Inputs=|+-
  Sum2 : Sum  Inputs=|+-
  Sum3 : Sum  Inputs=|+-
  Temperature Correct Pitch : Subsystem  Commented=through
  Temperature Correct Pitch1 : Subsystem
  Temperature Correct Roll : Subsystem  Commented=through
  Temperature Correct Roll1 : Subsystem
  Temperature Correct Yaw : Subsystem  Commented=through
  Temperature Correct Yaw1 : Subsystem
  Temperature Correct Yaw2 : Subsystem
  Calibrated-BodyRates : Outport
  wires:
  Discrete-Time Integrator/1 -> Drift Integration/1
  Bit Step to Deg/s/1 -> Discrete-Time Integrator/1
  Mux/1 -> Data Type Conversion/1, Bit Step to Deg/s/1
  Temperature Correct Yaw2/1(Offset Correct) -> Sum3/2
  Temperature Correct Pitch1/1(Offset Correct) -> Sum2/2
  Temperature Correct Roll1/1(Offset Correct) -> Sum1/2
  Convert to Celcius/1(Out1) -> Temperature Correct Roll/1(Temp), Temperature Correct Pitch/1(Temp), Temperature Correct Yaw/1(Temp)
  TempMeasure/1 -> Convert to Celcius/1(In1)
  Temperature Correct Yaw/1(Offset Correct) -> Temperature Correct Yaw1/1(Temp), Temperature Correct Yaw2/1(Temp)
  Temperature Correct Pitch/1(Offset Correct) -> Temperature Correct Pitch1/1(Temp)
  Temperature Correct Roll/1(Offset Correction) -> Temperature Correct Roll1/1(Temp)
  Mux3/1 -> Scope/3
  Mux2/1 -> Scope/2
  Mux1/1 -> Scope/1
  Sum2/1 -> Mux/2, Mux2/2  "Corrected Wy"
  Data Type Conversion/1 -> Calibrated-BodyRates/1
  PQR-Body Rates/1 -> Demux/1
  Demux/1 -> Sum1/1, Mux1/1  "Uncorrected Wx"
  Sum1/1 -> Mux/1, Mux1/2  "Corrected Wx"
  Demux/3 -> Sum3/1, Mux3/1  "Uncorrected Wz"
  Demux/2 -> Sum2/1, Mux2/1  "Uncorrected Wy"
  Sum3/1 -> Mux/3, Mux3/2  "Corrected Wz"

== system Navigation_Lib/Navigation Subsystem/SL3D Visualization/Interchange Axes Accel for SL3D  ==
  VRML_in : Inport
  Demux1 : Demux  Outputs=3
  Gain1 : Gain  Gain=3
  Gain2 : Gain
  Gain3 : Gain
  Mux2 : Mux  Inputs=3
  VRML_out : Outport
  wires:
  VRML_in/1 -> Gain1/1
  Demux1/2 -> Gain2/1
  Mux2/1 -> VRML_out/1
  Gain3/1 -> Mux2/3
  Gain2/1 -> Mux2/1
  Demux1/3 -> Mux2/2
  Demux1/1 -> Gain3/1
  Gain1/1 -> Demux1/1

== system Navigation_Lib/Navigation Subsystem/SL3D Visualization/Interchange Axes Mag for SL3D  ==
  VRML_in : Inport
  Home Drone : Subsystem
  Subsystem : Subsystem  Commented=on
  Work Drone : Subsystem
  Work Drone - supposed work drone .. not really : Subsystem
  VRML_out : Outport
  wires:
  Work Drone/1(Out1) -> VRML_out/1
  VRML_in/1 -> Home Drone/1(In1), Work Drone/1(In1)

== system Navigation_Lib/Navigation Subsystem/SL3D Visualization/Interchange Axis Mag Project for SL3D ==
  VRML_in : Inport
  Demux1 : Demux  Outputs=3
  Gain2 : Gain
  Gain3 : Gain
  Mux2 : Mux  Inputs=3
  VRML_out : Outport
  wires:
  Demux1/2 -> Gain2/1
  Mux2/1 -> VRML_out/1
  Gain3/1 -> Mux2/3
  Gain2/1 -> Mux2/1
  Demux1/3 -> Mux2/2
  Demux1/1 -> Gain3/1
  VRML_in/1 -> Demux1/1

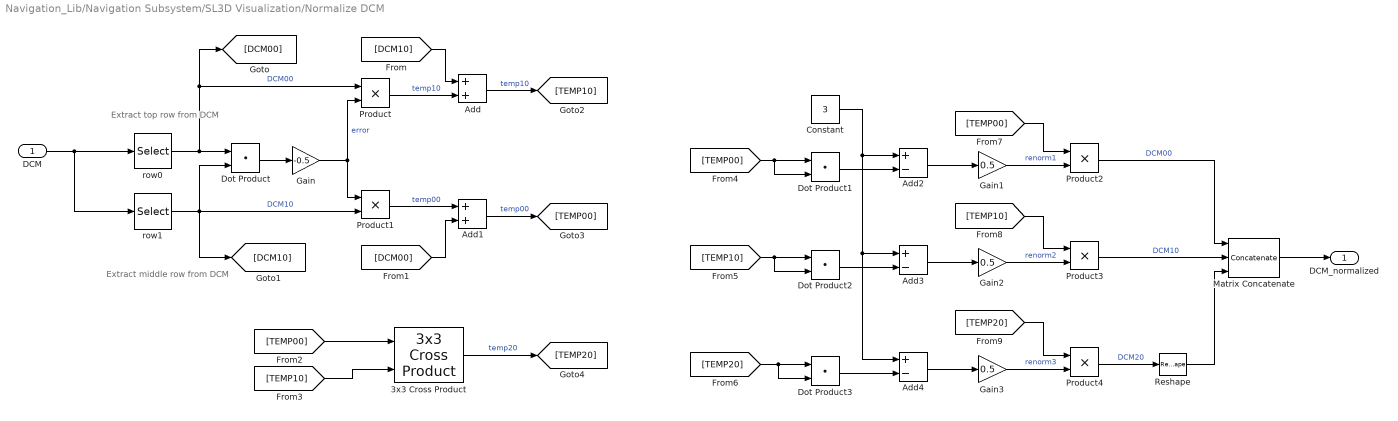
== system Navigation_Lib/Navigation Subsystem/SL3D Visualization/Normalize DCM ==
  note: Extract top row from DCM
  note: Extract middle row from DCM
  DCM : Inport  OutDataTypeStr=double  PortDimensions=[3,3]
  3x3 Cross Product : aerolibutil/3x3 Cross Product
  Add : Sum
  Add1 : Sum
  Add2 : Sum  Inputs=+-
  Add3 : Sum  Inputs=+-
  Add4 : Sum  Inputs=+-
  Constant : Constant  Value=3  OutDataTypeStr=double  SampleTime=-1
  Dot Product{,1..3} (4 alike) : DotProduct  InputSameDT=on  OutDataTypeStr=Inherit: Inherit via internal rule
  Gain : Gain  Gain=-0.5
  Gain1 : Gain  Gain=0.5  OutDataTypeStr=single
  Gain2 : Gain  Gain=0.5  OutDataTypeStr=single
  Gain3 : Gain  Gain=0.5  OutDataTypeStr=single
  Matrix Concatenate : Concatenate  NumInputs=3  Mode=Multidimensional array
  Product{,1..4} (5 alike) : Product  RndMeth=Zero
  Reshape : Reshape  OutputDimensionality=Row vector (2-D)
  row0 : Selector  NumberOfDimensions=2  IndexMode=Zero-based  InputPortWidth=3  IndexOptions=Index vector (dialog),Index vector (dialog)  Indices=0,[0:2]  OutputSizes=1,1
  row1 : Selector  NumberOfDimensions=2  IndexMode=Zero-based  InputPortWidth=3  IndexOptions=Index vector (dialog),Index vector (dialog)  Indices=1,[0:2]  OutputSizes=1,1
  DCM_normalized : Outport  OutDataTypeStr=double
  wires:
  DCM/1 -> row0/1, row1/1
  row0/1 -> Dot Product/1, Product/1, [DCM00]  "DCM00"
  row1/1 -> Dot Product/2, Product1/2, [DCM10]  "DCM10"
  Dot Product/1 -> Gain/1
  Gain/1 -> Product/2, Product1/1  "error"
  Product/1 -> Add/2  "temp10"
  Product1/1 -> Add1/1  "temp00"
  [DCM10] -> Add/1
  [DCM00] -> Add1/2
  Add/1 -> [TEMP10]  "temp10"
  Add1/1 -> [TEMP00]  "temp00"
  3x3 Cross Product/1 -> [TEMP20]  "temp20"
  [TEMP00] -> 3x3 Cross Product/1
  [TEMP10] -> 3x3 Cross Product/2
  [TEMP00] -> Dot Product1/1, Dot Product1/2
  [TEMP10] -> Dot Product2/1, Dot Product2/2
  [TEMP20] -> Dot Product3/1, Dot Product3/2
  Dot Product1/1 -> Add2/2
  Constant/1 -> Add2/1, Add4/1, Add3/1
  Add2/1 -> Gain1/1
  Gain1/1 -> Product2/2  "renorm1"
  Add3/1 -> Gain2/1
  Gain2/1 -> Product3/2  "renorm2"
  Dot Product2/1 -> Add3/2
  Add4/1 -> Gain3/1
  Gain3/1 -> Product4/2  "renorm3"
  Dot Product3/1 -> Add4/2
  [TEMP00] -> Product2/1
  [TEMP10] -> Product3/1
  [TEMP20] -> Product4/1
  Product2/1 -> Matrix Concatenate/1  "DCM00"
  Product3/1 -> Matrix Concatenate/2  "DCM10"
  Product4/1 -> Reshape/1  "DCM20"
  Matrix Concatenate/1 -> DCM_normalized/1
  Reshape/1 -> Matrix Concatenate/3

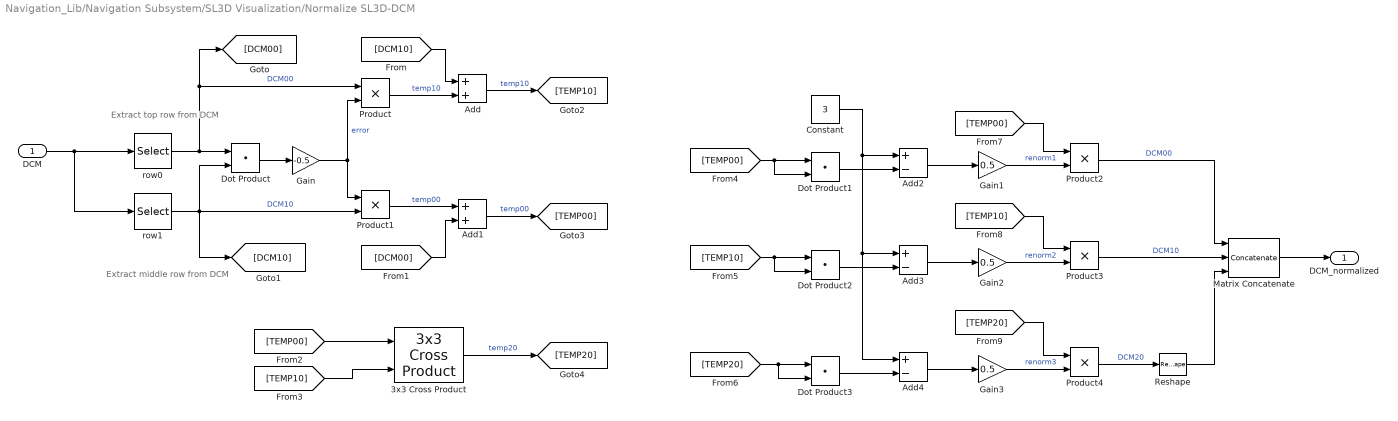
== system Navigation_Lib/Navigation Subsystem/SL3D Visualization/Normalize SL3D-DCM ==
  note: Extract top row from DCM
  note: Extract middle row from DCM
  DCM : Inport  OutDataTypeStr=double  PortDimensions=[3,3]
  3x3 Cross Product : aerolibutil/3x3 Cross Product
  Add : Sum
  Add1 : Sum
  Add2 : Sum  Inputs=+-
  Add3 : Sum  Inputs=+-
  Add4 : Sum  Inputs=+-
  Constant : Constant  Value=3  OutDataTypeStr=double  SampleTime=-1
  Dot Product{,1..3} (4 alike) : DotProduct  InputSameDT=on  OutDataTypeStr=Inherit: Inherit via internal rule
  Gain : Gain  Gain=-0.5
  Gain1 : Gain  Gain=0.5  OutDataTypeStr=single
  Gain2 : Gain  Gain=0.5  OutDataTypeStr=single
  Gain3 : Gain  Gain=0.5  OutDataTypeStr=single
  Matrix Concatenate : Concatenate  NumInputs=3  Mode=Multidimensional array
  Product{,1..4} (5 alike) : Product  RndMeth=Zero
  Reshape : Reshape  OutputDimensionality=Row vector (2-D)
  row0 : Selector  NumberOfDimensions=2  IndexMode=Zero-based  InputPortWidth=3  IndexOptions=Index vector (dialog),Index vector (dialog)  Indices=0,[0:2]  OutputSizes=1,1
  row1 : Selector  NumberOfDimensions=2  IndexMode=Zero-based  InputPortWidth=3  IndexOptions=Index vector (dialog),Index vector (dialog)  Indices=1,[0:2]  OutputSizes=1,1
  DCM_normalized : Outport  OutDataTypeStr=double
  wires:
  DCM/1 -> row0/1, row1/1
  row0/1 -> Dot Product/1, Product/1, [DCM00]  "DCM00"
  row1/1 -> Dot Product/2, Product1/2, [DCM10]  "DCM10"
  Dot Product/1 -> Gain/1
  Gain/1 -> Product/2, Product1/1  "error"
  Product/1 -> Add/2  "temp10"
  Product1/1 -> Add1/1  "temp00"
  [DCM10] -> Add/1
  [DCM00] -> Add1/2
  Add/1 -> [TEMP10]  "temp10"
  Add1/1 -> [TEMP00]  "temp00"
  3x3 Cross Product/1 -> [TEMP20]  "temp20"
  [TEMP00] -> 3x3 Cross Product/1
  [TEMP10] -> 3x3 Cross Product/2
  [TEMP00] -> Dot Product1/1, Dot Product1/2
  [TEMP10] -> Dot Product2/1, Dot Product2/2
  [TEMP20] -> Dot Product3/1, Dot Product3/2
  Dot Product1/1 -> Add2/2
  Constant/1 -> Add2/1, Add4/1, Add3/1
  Add2/1 -> Gain1/1
  Gain1/1 -> Product2/2  "renorm1"
  Add3/1 -> Gain2/1
  Gain2/1 -> Product3/2  "renorm2"
  Dot Product2/1 -> Add3/2
  Add4/1 -> Gain3/1
  Gain3/1 -> Product4/2  "renorm3"
  Dot Product3/1 -> Add4/2
  [TEMP00] -> Product2/1
  [TEMP10] -> Product3/1
  [TEMP20] -> Product4/1
  Product2/1 -> Matrix Concatenate/1  "DCM00"
  Product3/1 -> Matrix Concatenate/2  "DCM10"
  Product4/1 -> Reshape/1  "DCM20"
  Matrix Concatenate/1 -> DCM_normalized/1
  Reshape/1 -> Matrix Concatenate/3

== system Navigation_Lib/Navigation Subsystem/SL3D Visualization/Re-align X-axis ==
  MagVector : Inport
  Demux1 : Demux  Outputs=3
  Gain : Gain
  Gain1 : Gain  Gain=-1
  Gain2 : Gain
  Mux2 : Mux  Inputs=3
  MagVectorOut : Outport
  wires:
  MagVector/1 -> Demux1/1
  Gain/1 -> Mux2/3
  Gain2/1 -> Mux2/2
  Gain1/1 -> Mux2/1
  Demux1/3 -> Gain/1
  Demux1/2 -> Gain2/1
  Demux1/1 -> Gain1/1
  Mux2/1 -> MagVectorOut/1

== system Navigation_Lib/Navigation Subsystem/SL3D Visualization/SL3D DCM Output - used to adjust axes to fit wit SL3D convention ==

== system Navigation_Lib/Navigation Subsystem/SL3D Visualization/Subsystem ==
  DCM : Inport
  MagVector : Inport  Port=2
  Compensate for Magnetic Declination (~60 degrees in Boston)_ : MATLAB Function  Commented=through  TreatAsAtomicUnit=on
  Compensate for Magnetic Declination (~60 degrees in Boston)_1 : MATLAB Function  TreatAsAtomicUnit=on
  EnlargeVectorAgain : Gain  Commented=through  Gain=3
  Transform MagVector from Body Frame to World Frame : Product  Multiplication=Matrix(*)
  Transform compensated magnetic vector into the  body frame : Product  Multiplication=Matrix(*)
  Transpose2 : dspmtrx3/Transpose  Hermitian=off  overflowFlag=off
  Projected Mag Vector (body frame) : Outport
  Projected Mag Vector (global frame) : Outport  Port=2
  wires:
  Compensate for Magnetic Declination (~60 degrees in Boston)_1/1(y) -> Transform compensated magnetic vector into the  body frame/2, Projected Mag Vector (global frame)/1
  Compensate for Magnetic Declination (~60 degrees in Boston)_/1(y) -> Compensate for Magnetic Declination (~60 degrees in Boston)_1/1(vector_in)
  Transform MagVector from Body Frame to World Frame/1 -> Compensate for Magnetic Declination (~60 degrees in Boston)_/1(vector_in)
  Transpose2/1 -> Transform compensated magnetic vector into the  body frame/1
  EnlargeVectorAgain/1 -> Transform MagVector from Body Frame to World Frame/2
  DCM/1 -> Transform MagVector from Body Frame to World Frame/1, Transpose2/1
  Transform compensated magnetic vector into the  body frame/1 -> Projected Mag Vector (body frame)/1
  MagVector/1 -> EnlargeVectorAgain/1

== system Navigation_Lib/Navigation Subsystem/Attitude Determination/Calculate DCM/Calculate Deltas ==
  note: This needs to be investigated to see
      | if we can replace this with an actual
      | call to intrinsic timers to get the actual
      | elapsed time.
  Adjusted : Inport
  DriftCorrection : Inport  Port=2
  Add1 : Sum
  Add2 : Sum
  Constant : Constant  Value=1/400  SampleTime=-1
  Demux : Demux  Outputs=[3 3]
  Demux1 : Demux  Outputs=3
  Demux2 : Demux  Outputs=3
  Gain : Gain
  Gain1 : Gain
  Low Pass Filter1 : Subsystem
      mask Display: disp(['Elliptic Filter with 20 Hz corner', '\n', '44 dB stopband.'])
  Mux : Mux  Inputs=3
  Mux1 : Mux  Inputs=3
  Product1 : Product  RndMeth=Zero
  Gyro_Vector(G_Dt) : Outport
  Omega : Outport  Port=2
  wires:
  Constant/1 -> Product1/1  "DeltaT"
  Product1/1 -> Gyro_Vector(G_Dt)/1
  Low Pass Filter1/1(Output) -> Add1/2  "Gyro_Vector"
  Adjusted/1 -> Low Pass Filter1/1(Input)  "Gyro_Vector"
  DriftCorrection/1 -> Demux/1
  Add1/1 -> Add2/2
  Add2/1 -> Omega/1, Product1/2
  Demux/2 -> Demux1/1  "Omega_I"
  Demux/1 -> Demux2/1  "Omeg_P"
  Demux1/1 -> Mux/1
  Demux1/2 -> Mux/2
  Demux1/3 -> Gain/1
  Gain/1 -> Mux/3
  Mux/1 -> Add1/1
  Demux2/1 -> Mux1/1
  Demux2/2 -> Mux1/2
  Demux2/3 -> Gain1/1
  Gain1/1 -> Mux1/3
  Mux1/1 -> Add2/1

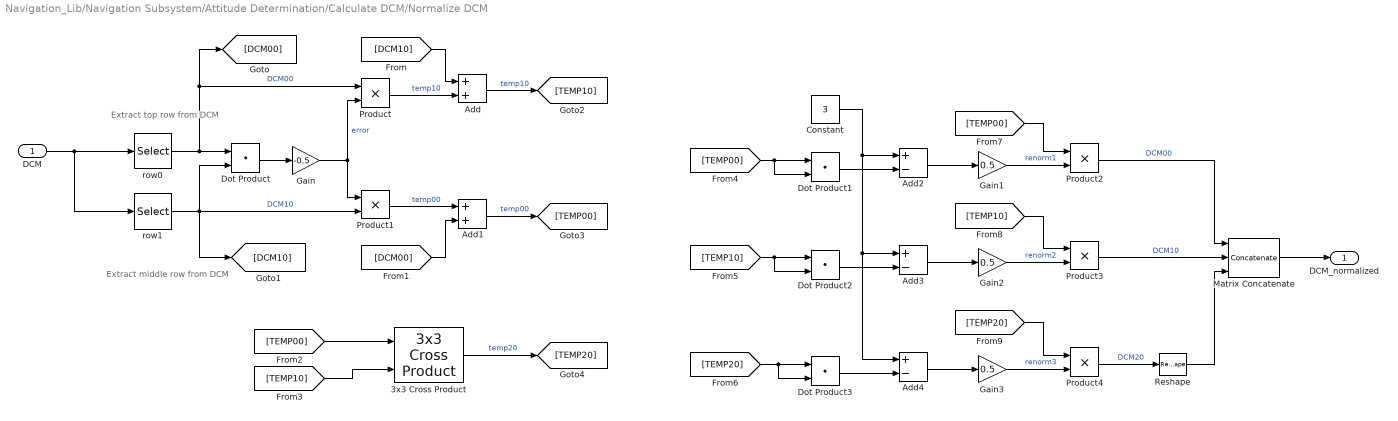
== system Navigation_Lib/Navigation Subsystem/Attitude Determination/Calculate DCM/Normalize DCM ==
  note: Extract middle row from DCM
  note: Extract top row from DCM
  DCM : Inport  OutDataTypeStr=double  PortDimensions=[3,3]
  3x3 Cross Product : aerolibutil/3x3 Cross Product
  Add : Sum
  Add1 : Sum
  Add2 : Sum  Inputs=+-
  Add3 : Sum  Inputs=+-
  Add4 : Sum  Inputs=+-
  Constant : Constant  Value=3  OutDataTypeStr=double  SampleTime=-1
  Dot Product{,1..3} (4 alike) : DotProduct  InputSameDT=on  OutDataTypeStr=Inherit: Inherit via internal rule
  Gain : Gain  Gain=-0.5
  Gain1 : Gain  Gain=0.5  OutDataTypeStr=single
  Gain2 : Gain  Gain=0.5  OutDataTypeStr=single
  Gain3 : Gain  Gain=0.5  OutDataTypeStr=single
  Matrix Concatenate : Concatenate  NumInputs=3  Mode=Multidimensional array
  Product{,1..4} (5 alike) : Product  RndMeth=Zero
  Reshape : Reshape  OutputDimensionality=Row vector (2-D)
  row0 : Selector  NumberOfDimensions=2  IndexMode=Zero-based  InputPortWidth=3  IndexOptions=Index vector (dialog),Index vector (dialog)  Indices=0,[0:2]  OutputSizes=1,1
  row1 : Selector  NumberOfDimensions=2  IndexMode=Zero-based  InputPortWidth=3  IndexOptions=Index vector (dialog),Index vector (dialog)  Indices=1,[0:2]  OutputSizes=1,1
  DCM_normalized : Outport  OutDataTypeStr=double
  wires:
  Reshape/1 -> Matrix Concatenate/3
  Matrix Concatenate/1 -> DCM_normalized/1
  Product4/1 -> Reshape/1  "DCM20"
  Product3/1 -> Matrix Concatenate/2  "DCM10"
  Product2/1 -> Matrix Concatenate/1  "DCM00"
  [TEMP20] -> Product4/1
  [TEMP10] -> Product3/1
  [TEMP00] -> Product2/1
  Dot Product3/1 -> Add4/2
  Gain3/1 -> Product4/2  "renorm3"
  Add4/1 -> Gain3/1
  Dot Product2/1 -> Add3/2
  Gain2/1 -> Product3/2  "renorm2"
  Add3/1 -> Gain2/1
  Gain1/1 -> Product2/2  "renorm1"
  Add2/1 -> Gain1/1
  Constant/1 -> Add3/1, Add4/1, Add2/1
  Dot Product1/1 -> Add2/2
  [TEMP20] -> Dot Product3/2, Dot Product3/1
  [TEMP10] -> Dot Product2/2, Dot Product2/1
  [TEMP00] -> Dot Product1/2, Dot Product1/1
  [TEMP10] -> 3x3 Cross Product/2
  [TEMP00] -> 3x3 Cross Product/1
  3x3 Cross Product/1 -> [TEMP20]  "temp20"
  Add1/1 -> [TEMP00]  "temp00"
  Add/1 -> [TEMP10]  "temp10"
  [DCM00] -> Add1/2
  [DCM10] -> Add/1
  Product1/1 -> Add1/1  "temp00"
  Product/1 -> Add/2  "temp10"
  Gain/1 -> Product1/1, Product/2  "error"
  Dot Product/1 -> Gain/1
  row1/1 -> [DCM10], Product1/2, Dot Product/2  "DCM10"
  row0/1 -> [DCM00], Product/1, Dot Product/1  "DCM00"
  DCM/1 -> row1/1, row0/1

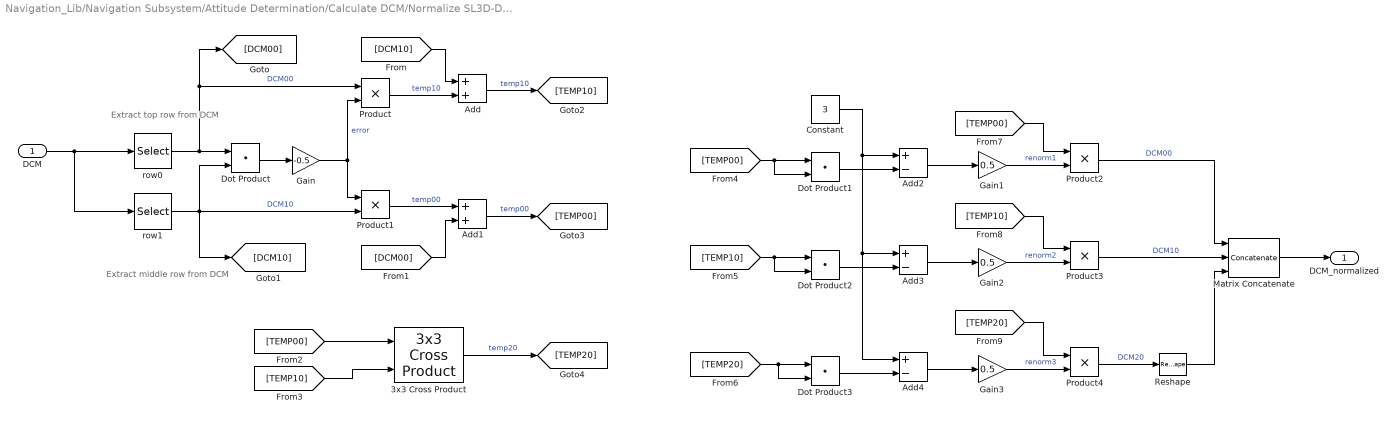
== system Navigation_Lib/Navigation Subsystem/Attitude Determination/Calculate DCM/Normalize SL3D-DCM ==
  note: Extract middle row from DCM
  note: Extract top row from DCM
  DCM : Inport  OutDataTypeStr=double  PortDimensions=[3,3]
  3x3 Cross Product : aerolibutil/3x3 Cross Product
  Add : Sum
  Add1 : Sum
  Add2 : Sum  Inputs=+-
  Add3 : Sum  Inputs=+-
  Add4 : Sum  Inputs=+-
  Constant : Constant  Value=3  OutDataTypeStr=double  SampleTime=-1
  Dot Product{,1..3} (4 alike) : DotProduct  InputSameDT=on  OutDataTypeStr=Inherit: Inherit via internal rule
  Gain : Gain  Gain=-0.5
  Gain1 : Gain  Gain=0.5  OutDataTypeStr=single
  Gain2 : Gain  Gain=0.5  OutDataTypeStr=single
  Gain3 : Gain  Gain=0.5  OutDataTypeStr=single
  Matrix Concatenate : Concatenate  NumInputs=3  Mode=Multidimensional array
  Product{,1..4} (5 alike) : Product  RndMeth=Zero
  Reshape : Reshape  OutputDimensionality=Row vector (2-D)
  row0 : Selector  NumberOfDimensions=2  IndexMode=Zero-based  InputPortWidth=3  IndexOptions=Index vector (dialog),Index vector (dialog)  Indices=0,[0:2]  OutputSizes=1,1
  row1 : Selector  NumberOfDimensions=2  IndexMode=Zero-based  InputPortWidth=3  IndexOptions=Index vector (dialog),Index vector (dialog)  Indices=1,[0:2]  OutputSizes=1,1
  DCM_normalized : Outport  OutDataTypeStr=double
  wires:
  Reshape/1 -> Matrix Concatenate/3
  Matrix Concatenate/1 -> DCM_normalized/1
  Product4/1 -> Reshape/1  "DCM20"
  Product3/1 -> Matrix Concatenate/2  "DCM10"
  Product2/1 -> Matrix Concatenate/1  "DCM00"
  [TEMP20] -> Product4/1
  [TEMP10] -> Product3/1
  [TEMP00] -> Product2/1
  Dot Product3/1 -> Add4/2
  Gain3/1 -> Product4/2  "renorm3"
  Add4/1 -> Gain3/1
  Dot Product2/1 -> Add3/2
  Gain2/1 -> Product3/2  "renorm2"
  Add3/1 -> Gain2/1
  Gain1/1 -> Product2/2  "renorm1"
  Add2/1 -> Gain1/1
  Constant/1 -> Add3/1, Add4/1, Add2/1
  Dot Product1/1 -> Add2/2
  [TEMP20] -> Dot Product3/2, Dot Product3/1
  [TEMP10] -> Dot Product2/2, Dot Product2/1
  [TEMP00] -> Dot Product1/2, Dot Product1/1
  [TEMP10] -> 3x3 Cross Product/2
  [TEMP00] -> 3x3 Cross Product/1
  3x3 Cross Product/1 -> [TEMP20]  "temp20"
  Add1/1 -> [TEMP00]  "temp00"
  Add/1 -> [TEMP10]  "temp10"
  [DCM00] -> Add1/2
  [DCM10] -> Add/1
  Product1/1 -> Add1/1  "temp00"
  Product/1 -> Add/2  "temp10"
  Gain/1 -> Product1/1, Product/2  "error"
  Dot Product/1 -> Gain/1
  row1/1 -> [DCM10], Product1/2, Dot Product/2  "DCM10"
  row0/1 -> [DCM00], Product/1, Dot Product/1  "DCM00"
  DCM/1 -> row1/1, row0/1

== system Navigation_Lib/Navigation Subsystem/Attitude Determination/Calculate DCM/Process Raw Rate Gyro Data ==
  note: const float Sensitivity[ 3 ] = { 0.0609 , 0.0609 , 0.0609 } ;
      | const float Neutral[ 3 ] = { 0.0 , 0.0 , 0.0 } ;
      | const int16_t Offset[ 3 ] = { - 73 , 14 , - 13 } ;
      | const int16_t Noises[ 3 ] = { 35 , 35 , 15 } ;
      |
      | int16_t vRaws[ 3 ] = {
      | Navdata :: IMU :: Gyroscope :: getRawX (),
      | Navdata :: IMU :: Gyroscope :: getRawY (),
      | Navdata :: IMU :: Gyroscope :: getRawZ ()
      | } ;
      |
      | gyroscope[i] = vRaws[i] * Gyroscope :: Sensitivity[i] * M_PI / 180.0 ;
  Raw Data : Inport
  Constant1 : Constant  Commented=on  Value=[gyro_x_offset, gyro_y_offset, gyro_z_offset]
  Gain : Gain  Gain=[0.0609, 0.0609, 0.0609*1]
  Sum : Sum  Inputs=|++
  Processed Data : Outport
  wires:
  Sum/1 -> Gain/1
  Gain/1 -> Processed Data/1
  Raw Data/1 -> Sum/1
  Constant1/1 -> Sum/2

== system Navigation_Lib/Navigation Subsystem/Attitude Determination/Calculate DCM/SL3D DCM Output - used to adjust axes to fit wit SL3D convention ==
